simulink library "PPT"  (R2016b)
settings: Solver=VariableStepAuto  StartTime=0.0  StopTime=10.0  RelTol=1e-3
undefined symbols (not defined in the file): sim_params
libraries: simulink x1
settings Model: Creator=scrice  LastModifiedBy=Taylor

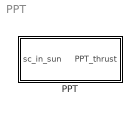
== system PPT ==
  PPT : Subsystem

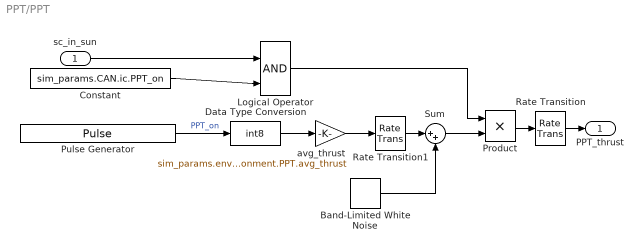
== system PPT/PPT ==
  sc_in_sun : Inport
  Band-Limited White Noise : simulink/Sources/Band-Limited White Noise  Cov=[0.1e-11]  Ts=sim_params.sample_time_s  seed=[23341]
  Constant : Constant  Value=sim_params.CAN.ic.PPT_on  SampleTime=sim_params.sample_time_s
  Data Type Conversion : DataTypeConversion  OutDataTypeStr=int8
  Logical Operator : Logic  IconShape=distinctive  AllPortsSameDT=off  OutDataTypeStr=boolean
  Product : Product
  Pulse Generator : DiscretePulseGenerator  PulseType=Time based  Period=sim_params.CAN.sync_pulse_period_s  PulseWidth=sim_params.actuators.ppt.t_on_pct
  Rate Transition : RateTransition
  Rate Transition1 : RateTransition
  Sum : Sum  Inputs=|++
  avg_thrust : Gain  Gain=sim_params.environment.PPT.avg_thrust
  PPT_thrust : Outport
  wires:
  Data Type Conversion/1 -> avg_thrust/1
  Pulse Generator/1 -> Data Type Conversion/1  "PPT_on"
  Band-Limited White Noise/1 -> Sum/2
  avg_thrust/1 -> Rate Transition1/1
  sc_in_sun/1 -> Logical Operator/1
  Constant/1 -> Logical Operator/2
  Logical Operator/1 -> Product/1
  Product/1 -> Rate Transition/1
  Sum/1 -> Product/2
  Rate Transition/1 -> PPT_thrust/1
  Rate Transition1/1 -> Sum/1
